simulink model "Copy_of_Simulink_Pendulum_Control_Offline"  (R2022b)
settings: Solver=ode1  StartTime=0.0  StopTime=20  FixedStep=0.001  RelTol=1e-3
undefined symbols (not defined in the file or in its folder): A, A_kf, alpha_max, B_kf, B_u, C_full, C_kf, D_full_u, D_kf, id_param, K_lq_en_alpha_eta_down, K_lq_en_alpha_x_down, L_p, sigbuilder_block, theta_max, voltage_max, x0, x0_ob
settings Model: Creator=utente  LastModifiedBy=federicocorso
settings SolverCC: AlgebraicLoopSolver=TrustRegion
settings DebuggingCC: UnconnectedInputMsg=warning  UnconnectedOutputMsg=warning  UnconnectedLineMsg=warning  SFMachineParentedDataDiag=warning
settings ModelReferenceCC: EnableRefExpFcnMdlSchedulingChecks=on

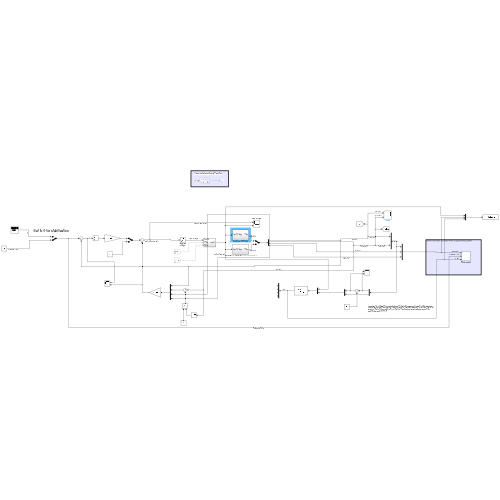
[thumbnail: Simulink's stored preview of the top-level diagram]
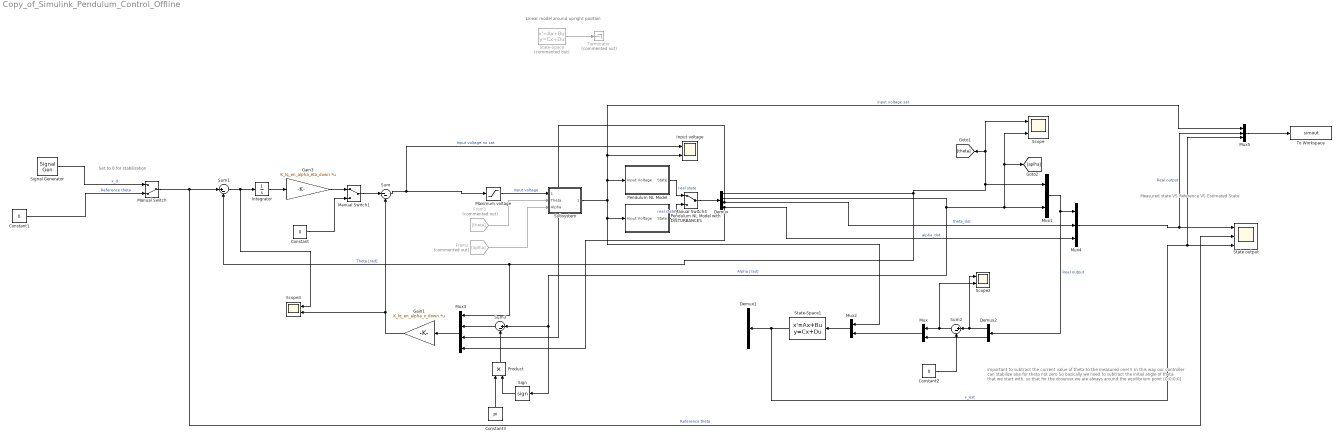
== system Copy_of_Simulink_Pendulum_Control_Offline ==
  note: Linear model around upright position
  note: important to subtract the current value of theta to the measured one!!! In this way our controller can stabilize also for theta not zero So basically we need to subtract the initial angle of theta that we start with, so that for the observer we are always around the equilibrium point [0;0;0;0]
  note: Measured state VS Reference VS Estimated State
  note: Set to 0 for stabilization
  Constant : Constant  Value=0
  Constant1 : Constant  Value=0
  Constant2 : Constant  Value=0
  Constant3 : Constant  Value=pi
  Demux : Demux
  Demux1 : Demux
  Demux2 : Demux  Outputs=2
  From1 : From  Commented=on  GotoTag=theta
  From2 : From  Commented=on  GotoTag=aplha
  Gain1 : Gain  Gain=K_lq_en_alpha_x_down  Multiplication=Matrix(K*u) (u vector)
  Gain3 : Gain  Gain=K_lq_en_alpha_eta_down  Multiplication=Matrix(K*u) (u vector)
  Input voltage : Scope  NumInputPorts=2
  Integrator : Integrator  LimitOutput=on  UpperSaturationLimit=3  LowerSaturationLimit=-3
  Manual Switch : ManualSwitch  CurrentSetting=0
  Manual Switch1 : ManualSwitch
  Manual Switch4 : ManualSwitch
  Maximum voltage : Saturate  UpperLimit=voltage_max  LowerLimit=-voltage_max
  Mux : Mux  Inputs=2
  Mux1 : Mux  Inputs=2
  Mux2 : Mux  Inputs=2
  Mux3 : Mux
  Mux4 : Mux  Inputs=3
  Mux5 : Mux  Inputs=3
  Pendulum NL Model : Subsystem
  Pendulum NL Model with DISTURBANCES : Subsystem
  Product : Product
  Scope : Scope  NumInputPorts=2
  Scope2 : Scope  NumInputPorts=2
  Scope3 : Scope  NumInputPorts=2
  Sign : Signum
  Signal Generator : SignalGenerator  WaveForm=square  Amplitude=0.3  Frequency=0.1
  State output : Scope  NumInputPorts=3
  State-Space : StateSpace  Commented=on  A=A  B=B_u  C=C_full  D=D_full_u  InitialCondition=x0
  State-Space1 : StateSpace  A=A_kf  B=B_kf  C=C_kf  D=D_kf  InitialCondition=x0_ob
  Subsystem : Subsystem
  Sum : Sum  Inputs=|--
  Sum1 : Sum  Inputs=|+-
  Sum2 : Sum  Inputs=|+-
  Sum3 : Sum  Inputs=|+-
  Terminator : Terminator  Commented=on
  To Workspace : ToWorkspace  VariableName=simout  SaveFormat=Timeseries  SampleTime=-1
  wires:
  Constant/1 -> Manual Switch1/2
  Sum1/1 -> Scope3/1, Integrator/1
  Mux3/1 -> Gain1/1
  Integrator/1 -> Gain3/1
  Gain3/1 -> Manual Switch1/1
  Demux/2 -> Sign/1, Sum3/1, Mux1/2, [aplha], Scope/2  "Alpha [rad]"
  Mux2/1 -> State-Space1/1
  Demux/1 -> Mux1/1, Scope/1, [theta], Mux3/1, Sum1/2  "Theta [rad]"
  From2/1 -> Subsystem/3(Alpha)
  From1/1 -> Subsystem/2(Theta)
  Subsystem/1(control) -> Pendulum NL Model/1(Input Voltage), Input voltage/2, Mux5/1, Pendulum NL Model with DISTURBANCES/1(Input Voltage), Mux2/1  "Input voltage sat"
  Gain1/1 -> Sum/2, Scope3/2
  Manual Switch/1 -> State output/2, Sum1/1  "Reference theta"
  Mux1/1 -> Demux2/1, Mux4/1  "Real output"
  Constant1/1 -> Manual Switch/2  "Reference theta"
  Signal Generator/1 -> Manual Switch/1  "x_d"
  Sum/1 -> Maximum voltage/1, Input voltage/1  "Input voltage no sat"
  State-Space1/1 -> Demux1/1, Mux5/3, State output/3  "x_est"
  Maximum voltage/1 -> Subsystem/1(Control)  "Input voltage"
  Manual Switch1/1 -> Sum/1
  State-Space/1 -> Terminator/1
  Demux/3 -> Mux3/3, Mux4/2  "theta_dot"
  Demux/4 -> Mux3/4, Mux4/3  "alpha_dot"
  Mux4/1 -> Mux5/2, State output/1  "Real output"
  Manual Switch4/1 -> Demux/1
  Pendulum NL Model/1(State) -> Manual Switch4/1  "real state"
  Mux/1 -> Mux2/2
  Demux2/2 -> Mux/2
  Demux2/1 -> Scope2/1, Sum2/1
  Sum2/1 -> Scope2/2, Mux/1
  Constant2/1 -> Sum2/2
  Mux5/1 -> To Workspace/1
  ? -> State-Space/1
  Pendulum NL Model with DISTURBANCES/1(State) -> Manual Switch4/2  "real state"
  Sum3/1 -> Mux3/2
  Constant3/1 -> Product/1
  Sign/1 -> Product/2
  Product/1 -> Sum3/2

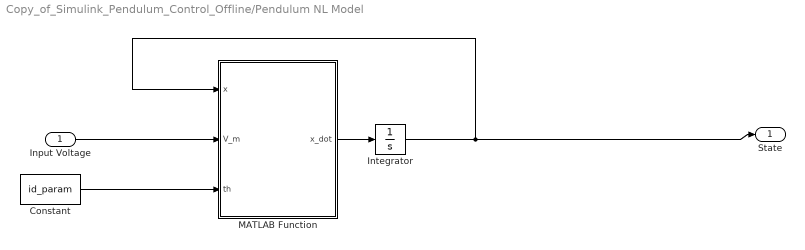
== system Copy_of_Simulink_Pendulum_Control_Offline/Pendulum NL Model ==
  Input Voltage : Inport
  Constant : Constant  Value=id_param
  Integrator : Integrator  InitialCondition=[1;-pi;0;0]
  MATLAB Function : MATLAB Function  TreatAsAtomicUnit=on
  State : Outport
  wires:
  Input Voltage/1 -> MATLAB Function/2(V_m)
  Constant/1 -> MATLAB Function/3(th)
  MATLAB Function/1(x_dot) -> Integrator/1
  Integrator/1 -> MATLAB Function/1(x), State/1

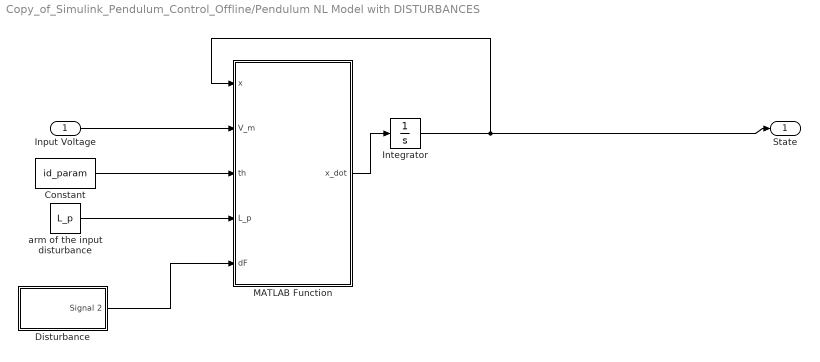
== system Copy_of_Simulink_Pendulum_Control_Offline/Pendulum NL Model with DISTURBANCES ==
  Input Voltage : Inport
  Constant : Constant  Value=id_param
  Disturbance : Subsystem  Tag=STV Subsys  LoadFcn=sigbuilder_block('load');  StartFcn=sigbuilder_block('start');  StopFcn=sigbuilder_block('stop');  ClipboardFcn=sigbuilder_block('clipboard');  mask(Sigbuilder block){tuvar=[0:10]}
      mask help: Simulink:masks:SigbuilderBlock_MD
      mask init:
      | if ~strcmp(get_param(bdroot(gcbh),'SimulationStatus'),'stopped') tuvar = sigbuilder_block('maskInit'); end
      settings: CopyFcn=sigbuilder_block('copy');  DeleteFcn=sigbuilder_block('delete');  ModelCloseFcn=sigbuilder_block('modelClose');  PreSaveFcn=sigbuilder_block('preSave');  PauseFcn=sigbuilder_block('pause');  ContinueFcn=sigbuilder_block('continue');  NameChangeFcn=sigbuilder_block('namechange');  OpenFcn=sigbuilder_block('open',[721 317 674 405 ]);  CloseFcn=sigbuilder_block('close');
      mask Display: plot(0, 0, 100, 100,[2, 2, 32, 32, 2], [68, 8, 8, 68, 68],[32, 2], [38, 38], [32, 19, 2],[53, 60, 44], [32, 17, 17, 2],[16, 16, 31, 31]);txt = getActiveGroup(gcbh);text(2, 100, txt,'verticalAlignment', 'top');
  Integrator : Integrator  InitialCondition=[0;0.15;0;0]
  MATLAB Function : MATLAB Function  TreatAsAtomicUnit=on
  arm of the input disturbance : Constant  Value=L_p
  State : Outport
  wires:
  Integrator/1 -> State/1, MATLAB Function/1(x)
  MATLAB Function/1(x_dot) -> Integrator/1
  Constant/1 -> MATLAB Function/3(th)
  Input Voltage/1 -> MATLAB Function/2(V_m)
  arm of the input disturbance/1 -> MATLAB Function/4(L_p)
  Disturbance/1(Signal 2) -> MATLAB Function/5(dF)

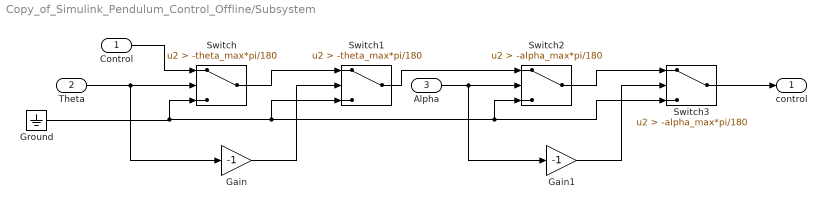
== system Copy_of_Simulink_Pendulum_Control_Offline/Subsystem ==
  Control : Inport
  Theta : Inport  Port=2
  Alpha : Inport  Port=3
  Gain : Gain  Gain=-1
  Gain1 : Gain  Gain=-1
  Ground : Ground
  Switch : Switch  Criteria=u2 > Threshold  Threshold=-theta_max*pi/180  SaturateOnIntegerOverflow=off  InputSameDT=off
  Switch1 : Switch  Criteria=u2 > Threshold  Threshold=-theta_max*pi/180  SaturateOnIntegerOverflow=off  InputSameDT=off
  Switch2 : Switch  Criteria=u2 > Threshold  Threshold=-alpha_max*pi/180  SaturateOnIntegerOverflow=off  InputSameDT=off
  Switch3 : Switch  Criteria=u2 > Threshold  Threshold=-alpha_max*pi/180  SaturateOnIntegerOverflow=off  InputSameDT=off
  control : Outport
  wires:
  Gain/1 -> Switch1/2
  Theta/1 -> Gain/1, Switch/2
  Control/1 -> Switch/1
  Switch/1 -> Switch1/1
  Gain1/1 -> Switch3/2
  Switch1/1 -> Switch2/1
  Ground/1 -> Switch3/3, Switch2/3, Switch1/3, Switch/3
  Switch2/1 -> Switch3/1
  Alpha/1 -> Switch2/2, Gain1/1
  Switch3/1 -> control/1

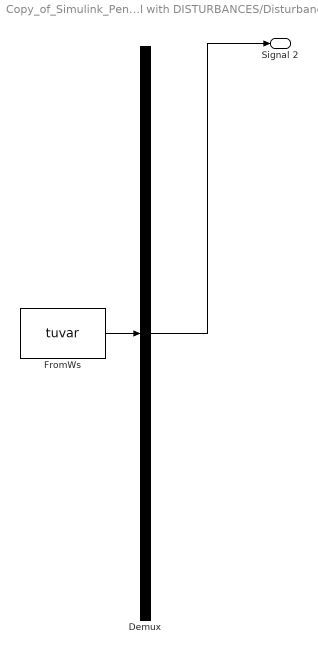
== system Copy_of_Simulink_Pendulum_Control_Offline/Pendulum NL Model with DISTURBANCES/Disturbance ==
  Demux : Demux  Tag=STV Demux  Outputs=1
      settings: DisplayOption=none
  FromWs : FromWorkspace  Tag=STV FromWs  VariableName=tuvar
      SigBuilderData=|
      | common.afterFinalStr = 'Extrapolate'
      | common.sampleTime = 0
      | dataSet.timeRange = [0 20]
      | dataSet.name = 'Group 1'
      | sbobj.Groups.Name = 'Group 1'
      | sbobj.Groups.Signals.Name = 'Signal 2'
      | sbobj.Groups.Signals.XData = [0 9.9 9.9 10 10 20]
      | sbobj.Groups.Signals.YData = [0 0 0.075 0.075 0 0]
      | sbobj.Groups.TimeRange = [0 20]
  Signal 2 : Outport  Tag=STV Outport
  wires:
  FromWs/1 -> Demux/1
  Demux/1 -> Signal 2/1

== matlab function Copy_of_Simulink_Pendulum_Control_Offline/Pendulum NL Model with DISTURBANCES/MATLAB Function ==
  data: x input; x_dot output; V_m input; th input; L_p input; dF input
function x_dot = NL_eqns_Disturbance(x,V_m,th,L_p,dF)
%NL_eqns_Disturbance
%    NL_DIFF_EQNS_SS = NL_eqns_Disturbance(B_p,B_r,J_a,J_p,M_d,G,L_P,M_P,R,TAU,x(2,1),x(3,1),x(4,1),x_dot(1,1),x_dot(2,1),x_dot(3,1),x_dot(4,1))

%    This function was generated by the Symbolic Math Toolbox version 9.2.
%    07-May-2023 08:47:27

B_p = th(1,1);
B_r = th(2,1);
J_a = th(3,1);
J_p = th(4,1);
l_p = th(5,1);
m_p = th(6,1);
r = th(7,1);
g = th(8,1);
K_g = th(9,1);
R_m = th(10,1);
eta_g = th(11,1);
eta_m = th(12,1);
k_m = th(13,1);
k_t = th(14,1);

tau = eta_g*K_g*eta_m*k_t*(V_m-K_g*k_m*x(3,1))/R_m; % motor torque expression-STATIC

M_d = L_p*dF; % moment of disturbance acting on alpha, where L_p is the position along the pendulum

t2 = cos(x(2,1));
t3 = sin(x(2,1));
t4 = l_p.^2;
t5 = l_p.^3;
t7 = m_p.^2;
t8 = r.^2;
t9 = x(2,1).*2.0;
t10 = x(3,1).^2;
t11 = x(4,1).^2;
t12 = J_a.*J_p;
t6 = t4.^2;
t13 = t2.^2;
t14 = sin(t9);
t15 = J_a.*m_p.*t4;
t16 = J_p.*m_p.*t4;
t17 = J_p.*m_p.*t8;
t20 = t4.*t7.*t8;
t18 = t6.*t7;
t19 = t13.*t16;
t24 = t13.*t20;
t21 = t13.*t18;
t22 = -t19;
t25 = -t24;
t23 = -t21;
t26 = t12+t15+t16+t17+t18+t20+t22+t23+t25;
t27 = 1.0./t26;

x_dot = zeros(4,1);

x_dot(1,1) = x(3,1);
x_dot(2,1) = x(4,1);
x_dot(3,1) = t27.*(J_p.*tau.*-2.0+B_r.*J_p.*x(3,1).*2.0-m_p.*t4.*tau.*2.0+t14.*t16.*x(3,1).*x(4,1).*2.0+t14.*t18.*x(3,1).*x(4,1).*2.0+B_r.*m_p.*t4.*x(3,1).*2.0-M_d.*l_p.*m_p.*r.*t2.*2.0+r.*t3.*t5.*t7.*t11.*2.0-g.*r.*t2.*t3.*t4.*t7.*2.0-r.*t2.*t5.*t7.*t10.*t14+B_p.*l_p.*m_p.*r.*t2.*x(4,1).*2.0+J_p.*l_p.*m_p.*r.*t3.*t11.*2.0).*(-1.0./2.0);
x_dot(4,1) = (t27.*(J_a.*M_d.*2.0-B_p.*J_a.*x(4,1).*2.0+M_d.*m_p.*t4.*2.0+M_d.*m_p.*t8.*2.0+t10.*t14.*t15+t10.*t14.*t18+t10.*t14.*t20+t10.*t14.*t23-M_d.*m_p.*t4.*t13.*2.0+g.*t3.*t5.*t7.*2.0-t2.*t3.*t11.*t20.*2.0-B_p.*m_p.*t4.*x(4,1).*2.0-B_p.*m_p.*t8.*x(4,1).*2.0+J_a.*g.*l_p.*m_p.*t3.*2.0+B_p.*m_p.*t4.*t13.*x(4,1).*2.0+g.*l_p.*t3.*t7.*t8.*2.0+l_p.*m_p.*r.*t2.*tau.*2.0-g.*t3.*t5.*t7.*t13.*2.0-B_r.*l_p.*m_p.*r.*t2.*x(3,1).*2.0-r.*t2.*t5.*t7.*t14.*x(3,1).*x(4,1).*2.0))./2.0;

== matlab function Copy_of_Simulink_Pendulum_Control_Offline/Pendulum NL Model/MATLAB Function ==
  data: x input; x_dot output; V_m input; th input
function x_dot = NL_eqns(x,V_m,th)
%NL_eqns
%    NL_DIFF_EQNS_SS = NL_eqns(B_p,B_r,J_a,J_p,G,L_P,M_P,R,TAU,x(2,1),x(3,1),x(4,1),X_DOT_1,X_DOT_2,X_DOT_3,X_DOT_4)

%    This function was generated by the Symbolic Math Toolbox version 9.2.
%    09-Mar-2023 15:34:15
B_p = th(1,1);
B_r = th(2,1);
J_a = th(3,1);
J_p = th(4,1);
l_p = th(5,1);
m_p = th(6,1);
r = th(7,1);
g = th(8,1);
K_g = th(9,1);
R_m = th(10,1);
eta_g = th(11,1);
eta_m = th(12,1);
k_m = th(13,1);
k_t = th(14,1);

tau = eta_g*K_g*eta_m*k_t*(V_m-K_g*k_m*x(3,1))/R_m; % motor torque expression-STATIC

t2 = cos(x(2,1));
t3 = sin(x(2,1));
t4 = l_p.^2;
t5 = l_p.^3;
t7 = m_p.^2;
t8 = r.^2;
t9 = x(2,1).*2.0;
t10 = x(3,1).^2;
t11 = x(4,1).^2;
t12 = J_a.*J_p;
t6 = t4.^2;
t13 = t2.^2;
t14 = sin(t9);
t15 = J_a.*m_p.*t4;
t16 = J_p.*m_p.*t4;
t17 = J_p.*m_p.*t8;
t20 = t4.*t7.*t8;
t18 = t6.*t7;
t19 = t13.*t16;
t24 = t13.*t20;
t21 = t13.*t18;
t22 = -t19;
t25 = -t24;
t23 = -t21;
t26 = t12+t15+t16+t17+t18+t20+t22+t23+t25;
t27 = 1.0./t26;

x_dot = zeros(4,1);

x_dot(1,1) = x(3,1);
x_dot(2,1) = x(4,1);
x_dot(3,1) = t27.*(J_p.*tau.*-2.0+B_r.*J_p.*x(3,1).*2.0-m_p.*t4.*tau.*2.0+t14.*t16.*x(3,1).*x(4,1).*2.0+t14.*t18.*x(3,1).*x(4,1).*2.0+B_r.*m_p.*t4.*x(3,1).*2.0+r.*t3.*t5.*t7.*t11.*2.0-g.*r.*t2.*t3.*t4.*t7.*2.0-r.*t2.*t5.*t7.*t10.*t14+B_p.*l_p.*m_p.*r.*t2.*x(4,1).*2.0+J_p.*l_p.*m_p.*r.*t3.*t11.*2.0).*(-1.0./2.0);
x_dot(4,1) = t27.*(B_p.*J_a.*x(4,1).*2.0-t10.*t14.*t15-t10.*t14.*t18-t10.*t14.*t20+t10.*t14.*t21-g.*t3.*t5.*t7.*2.0+t2.*t3.*t11.*t20.*2.0+B_p.*m_p.*t4.*x(4,1).*2.0+B_p.*m_p.*t8.*x(4,1).*2.0-J_a.*g.*l_p.*m_p.*t3.*2.0-B_p.*m_p.*t4.*t13.*x(4,1).*2.0-g.*l_p.*t3.*t7.*t8.*2.0-l_p.*m_p.*r.*t2.*tau.*2.0+g.*t3.*t5.*t7.*t13.*2.0+B_r.*l_p.*m_p.*r.*t2.*x(3,1).*2.0+r.*t2.*t5.*t7.*t14.*x(3,1).*x(4,1).*2.0).*(-1.0./2.0);

% x_plus_1 = zeros(4,1);
% x_plus_1 = x + Ts*x_dot;

% x_plus_1(1,1) = x(1,1) + Ts*x_dot(1,1);
% x_plus_1(1,1) = x(1,1) + Ts*x_dot(1,1);
% x_plus_1(1,1) = x(1,1) + Ts*x_dot(1,1);
% x_plus_1(1,1) = x(1,1) + Ts*x_dot(1,1);
